simulink library "DCDC_Converter"  (R2018b)
settings: Solver=VariableStepAuto  StartTime=0.0  StopTime=10.0  RelTol=1e-3
undefined symbols (not defined in the file): eff, Load
settings Model: Creator=Alexander Koch  LastModifiedBy=ga69qig
settings SFSimCC: SimUseLocalCustomCode=off
settings RTWCC: RTWUseLocalCustomCode=off
settings CodeAppCC: StateflowObjectComments=on

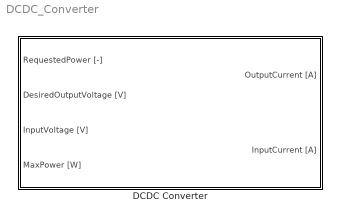
== system DCDC_Converter ==
  DCDC Converter : Subsystem  InitFcn=""  mask(SB){Pmax=4000, Umax=310, Umin=20, etaMax=0.97, etaDrop=0.03, LocalSampleTime=-1}
      mask prompts: Pmax "Maximal Power [W]"; Umax "Maximal Output Voltage [V]"; Umin "Minimal Input Voltage [V]"; etaMax "Maxinal Efficiency [-]"; etaDrop "Efficiency Drop at Maximal Ratio [-]"; LocalSampleTime "Local System Sample-Time [s]"
      mask help:
      | <Author> Alexander Koch based on Richard Eckl [1]</Author>
      | <Date> 03/04/2017 </Date>
      |
      | <Description>
      | Requires the requested power, desired output voltage, input voltage, maximal power of the energy supplier, max power of DCDC converter, maximal output voltage, minmal input voltage, maximal efficiency and the efficiency drop at maximal ratio. It calculates the output current which is at the desired output voltage and the input current which the energy suplier has to deliver.
      | Requested power is a value between 0 and 1. At 1, it delivers the maximal power of the energy supplier. If the input voltage drops unter the minmal input voltage, the current stops. This happens with a defined relay. Please check the relay block under the mask for further information. If the desired output voltage is higher than the maximal output voltage the simulation is forced to stop.
      | </Description>
      mask init:
      | GlobalSampleTime = CalcGlobalSampleTime(LocalSampleTime);
      | 
      | [eff, Load]=InitDCDCConverter()
      mask Help:
      | <Parameters>
      | Maximal Power [W]
      | 	<Min> 0 </Min>
      | Maximal Output Voltage [V]
      | 	<Min> 0 </Min>
      | Minimal Input Voltage [V]
      | Maximal Efficiency [-]
      | 	<Min> 0 </Min>
      | 	<Max> 1 </Max>
      | Efficiency Drop at Maximal Ratio [-]
      | 	<Min> 0 </Min>
      | 	<Max> Maximal Efficiency </Max>
      | Local System Sample-Time [s]
      | 	<Min> GlobalSampleTime </Min>
      | Global Sample-Time [s]
      | </Parameters>
      | 
      | <Inputs>
      | RequestedPower [-]
      | 	<Min> 0 </Min>
      | 	<Max> 1 </Max>
      | DesiredOutputVoltage [V]
      | 	<Min> 0 </Min>
      | InputVoltage [V]
      | 	<Min> 0 ? </Min>
      | MaxPower [W]
      | 	<Min> 0 </Min>
      | </Inputs>
      | 
      | <Outputs>
      | OutputCurrent [A]
      | InputCurrent [A]
      | </Outputs>
      | 
      | <Sources>
      | [1] R. Eckl, “Untersuchung und Bewertung von Technologien zur Reichweitensteigerung bei kleinen Elektrofahrzeugen,” Dissertation, Institute of Automotive Technology, Technical University Munich, 2016.
      | </Sources>
      mask TypeOptions Pmax: Saturation/UpperLimit | maxPower/Value
      mask TypeOptions Umax: Saturation1/UpperLimit | effDropByRatio/Umax/Value
      mask TypeOptions Umin: effDropByRatio/Umin/Value
      mask TypeOptions etaMax: max Wirkungsgrad/Gain
      mask TypeOptions etaDrop: effDropByRatio/etaDrop/Value
      mask TypeOptions LocalSampleTime: RequestedPower [-]/SampleTime | DesiredOutputVoltage [V]/SampleTime | InputVoltage [V]/SampleTime | MaxPower [W]/SampleTime
      mask DialogControl Container3 Prompt: Documentation:
      mask DialogControl DescHelpVar Prompt: %<MaskHelp>
      mask DialogControl Container5 Prompt: Sample Time
      mask Display:
      | [picturexpos,pictureypos,picturewidth,pictureheight] = ...
      |     CalcBlockPicturePosition(gcb,1,0.1,0.1,110,80); % calculating picture position depending on Block size and minimum margin size
      | image('DCDC_Converter.svg',[picturexpos pictureypos picturewidth pictureheight])% plot picture to block

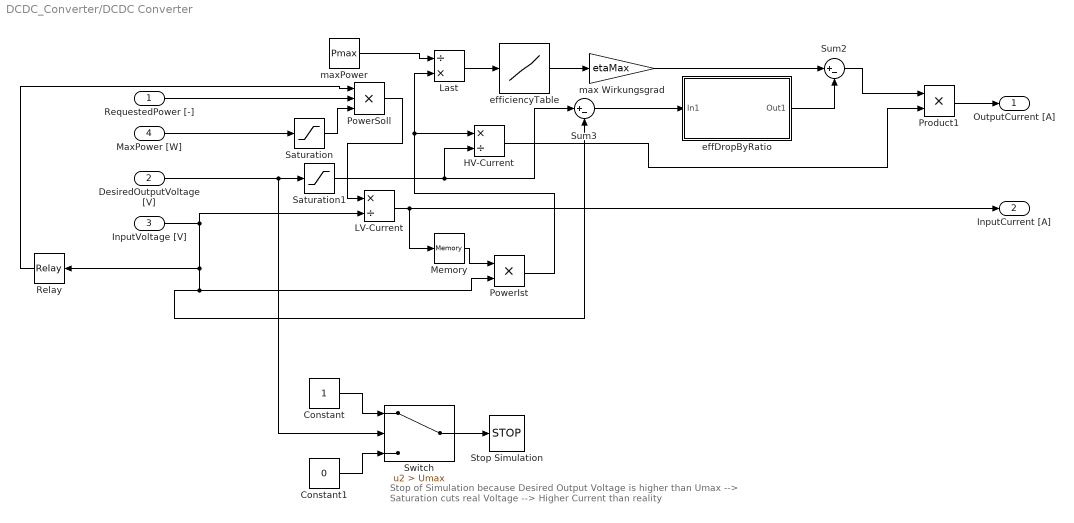
== system DCDC_Converter/DCDC Converter ==
  note: Stop of Simulation because Desired Output Voltage is higher than Umax
      | --> Saturation cuts real Voltage --> Higher Current than reality
  RequestedPower [-] : Inport  SampleTime=LocalSampleTime
  DesiredOutputVoltage [V] : Inport  Port=2  SampleTime=LocalSampleTime
  InputVoltage [V] : Inport  Port=3  SampleTime=LocalSampleTime
  MaxPower [W] : Inport  Port=4  SampleTime=LocalSampleTime
  Constant : Constant
  Constant1 : Constant  Value=0
  HV-Current : Product  Inputs=*/
  LV-Current : Product  Inputs=*/
  Last : Product  Inputs=/*
  Memory : Memory
  PowerIst : Product  RndMeth=Zero
  PowerSoll : Product  Inputs=3  RndMeth=Zero
  Product1 : Product
  Relay : Relay  OnSwitchValue=Umin+12  OffSwitchValue=Umin-3
  Saturation : Saturate  UpperLimit=Pmax  LowerLimit=0
  Saturation1 : Saturate  UpperLimit=Umax  LowerLimit=0
  Stop Simulation : Stop
  Sum2 : Sum  Inputs=|+-
  Sum3 : Sum  Inputs=|+-
  Switch : Switch  Criteria=u2 > Threshold  Threshold=Umax
  effDropByRatio : Subsystem
  efficiencyTable : Lookup_n-D  NumberOfTableDimensions=1  BreakpointsForDimension1=Load  Table=eff  RndMeth=Simplest  InputSameDT=on
  max Wirkungsgrad : Gain  Gain=etaMax
  maxPower : Constant  Value=Pmax
  OutputCurrent [A] : Outport  SampleTime=GlobalSampleTime
  InputCurrent [A] : Outport  Port=2  SampleTime=GlobalSampleTime
  wires:
  Memory/1 -> PowerIst/1
  InputVoltage [V]/1 -> LV-Current/2, Sum3/2, PowerIst/2, Relay/1
  PowerSoll/1 -> LV-Current/1
  LV-Current/1 -> Memory/1, InputCurrent [A]/1
  PowerIst/1 -> Last/2, HV-Current/1
  Sum2/1 -> Product1/1
  HV-Current/1 -> Product1/2
  Product1/1 -> OutputCurrent [A]/1
  effDropByRatio/1(Out1) -> Sum2/2
  Sum3/1 -> effDropByRatio/1(In1)
  Saturation/1 -> PowerSoll/3
  RequestedPower [-]/1 -> PowerSoll/2
  Relay/1 -> PowerSoll/1
  MaxPower [W]/1 -> Saturation/1
  maxPower/1 -> Last/1
  Last/1 -> efficiencyTable/1
  efficiencyTable/1 -> max Wirkungsgrad/1
  max Wirkungsgrad/1 -> Sum2/1
  Saturation1/1 -> Sum3/1, HV-Current/2
  Switch/1 -> Stop Simulation/1
  DesiredOutputVoltage [V]/1 -> Saturation1/1, Switch/2
  Constant/1 -> Switch/1
  Constant1/1 -> Switch/3

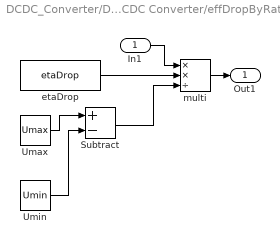
== system DCDC_Converter/DCDC Converter/effDropByRatio ==
  In1 : Inport
  Subtract : Sum  Inputs=+-
  Umax : Constant  Value=Umax
  Umin : Constant  Value=Umin
  etaDrop : Constant  Value=etaDrop
  multi : Product  Inputs=**/  RndMeth=Zero
  Out1 : Outport
  wires:
  Subtract/1 -> multi/3
  Umin/1 -> Subtract/2
  Umax/1 -> Subtract/1
  etaDrop/1 -> multi/2
  In1/1 -> multi/1
  multi/1 -> Out1/1
